simulink model "CPGPernaDireita"  (R2020a)
settings: Solver=VariableStepAuto  StartTime=0.0  StopTime=0.54  RelTol=1e-4
values from neighbouring files (symbols this model uses):
  b1 = 14.786    [CPG_PernaDireita_Parametros.m]
  b2 = b    (= 2.5)    [CPG_PernaDireita_Parametros.m]
  b3 = b    (= 2.5)    [CPG_PernaDireita_Parametros.m]
  b5 = b    (= 2.5)    [CPG_PernaDireita_Parametros.m]
  feed1 = 0    [CPG_PernaDireita_Parametros.m]
  feed10 = 0    [CPG_PernaDireita_Parametros.m]
  feed2 = 0    [CPG_PernaDireita_Parametros.m]
  feed3 = 0    [CPG_PernaDireita_Parametros.m]
  feed4 = 0    [CPG_PernaDireita_Parametros.m]
  feed5 = 0    [CPG_PernaDireita_Parametros.m]
  feed6 = 0    [CPG_PernaDireita_Parametros.m]
  feed9 = 0    [CPG_PernaDireita_Parametros.m]
  S1 = 50    [CPG_PernaDireita_Parametros.m]
  S2 = S0    (= 5)    [CPG_PernaDireita_Parametros.m]
  S3 = S0    (= 5)    [CPG_PernaDireita_Parametros.m]
  S5 = S0    (= 5)    [CPG_PernaDireita_Parametros.m]
  ta1 = 0.04    [CPG_PernaDireita_Parametros.m]
  ta10 = 0.3    [CPG_PernaDireita_Parametros.m]
  ta2 = 20    [CPG_PernaDireita_Parametros.m]
  ta3 = 0.6    [CPG_PernaDireita_Parametros.m]
  ta4 = 0.6    [CPG_PernaDireita_Parametros.m]
  ta5 = 0.3    [CPG_PernaDireita_Parametros.m]
  ta6 = 0.3    [CPG_PernaDireita_Parametros.m]
  ta9 = 0.3    [CPG_PernaDireita_Parametros.m]
  tr1 = 0.0004    [CPG_PernaDireita_Parametros.m]
  tr10 = 0.025    [CPG_PernaDireita_Parametros.m]
  tr2 = 0.1    [CPG_PernaDireita_Parametros.m]
  tr3 = 0.0005    [CPG_PernaDireita_Parametros.m]
  tr4 = 0.05    [CPG_PernaDireita_Parametros.m]
  tr5 = 0.025    [CPG_PernaDireita_Parametros.m]
  tr6 = 0.025    [CPG_PernaDireita_Parametros.m]
  tr9 = 0.025    [CPG_PernaDireita_Parametros.m]
  w10_1 = -1    [CPG_PernaDireita_Parametros.m]
  w10_2 = -1    [CPG_PernaDireita_Parametros.m]
  w10_5 = 0    [CPG_PernaDireita_Parametros.m]
  w10_6 = 0    [CPG_PernaDireita_Parametros.m]
  w10_9 = -2    [CPG_PernaDireita_Parametros.m]
  w12 = -2.64    [CPG_PernaDireita_Parametros.m]
  w13 = -1.7585    [CPG_PernaDireita_Parametros.m]
  w15 = 0    [CPG_PernaDireita_Parametros.m]
  w16 = 0    [CPG_PernaDireita_Parametros.m]
  w19 = 0    [CPG_PernaDireita_Parametros.m]
  w1_10 = 0    [CPG_PernaDireita_Parametros.m]
  w21 = -2    [CPG_PernaDireita_Parametros.m]
  w24 = -1    [CPG_PernaDireita_Parametros.m]
  w25 = 0    [CPG_PernaDireita_Parametros.m]
  w26 = 0    [CPG_PernaDireita_Parametros.m]
  w29 = 0    [CPG_PernaDireita_Parametros.m]
  w2_10 = 0    [CPG_PernaDireita_Parametros.m]
  w31 = -1    [CPG_PernaDireita_Parametros.m]
  w34 = -2    [CPG_PernaDireita_Parametros.m]
  w37 = 0    [CPG_PernaDireita_Parametros.m]
  w38 = 0    [CPG_PernaDireita_Parametros.m]
  w3_11 = 0    [CPG_PernaDireita_Parametros.m]
  w3_12 = 0    [CPG_PernaDireita_Parametros.m]
  w42 = -1    [CPG_PernaDireita_Parametros.m]
  w43 = -2    [CPG_PernaDireita_Parametros.m]
  w47 = 0    [CPG_PernaDireita_Parametros.m]
  w48 = 0    [CPG_PernaDireita_Parametros.m]
  w4_11 = 0    [CPG_PernaDireita_Parametros.m]
  w4_12 = 0    [CPG_PernaDireita_Parametros.m]
  w51 = 0    [CPG_PernaDireita_Parametros.m]
  w52 = 0    [CPG_PernaDireita_Parametros.m]
  w56 = -2    [CPG_PernaDireita_Parametros.m]
  w59 = 0    [CPG_PernaDireita_Parametros.m]
  w5_10 = 0    [CPG_PernaDireita_Parametros.m]
  w61 = -1    [CPG_PernaDireita_Parametros.m]
  w62 = -1    [CPG_PernaDireita_Parametros.m]
  w65 = -2    [CPG_PernaDireita_Parametros.m]
  w69 = 0    [CPG_PernaDireita_Parametros.m]
  w6_10 = 0    [CPG_PernaDireita_Parametros.m]
  w91 = 0    [CPG_PernaDireita_Parametros.m]
  w92 = 0    [CPG_PernaDireita_Parametros.m]
  w95 = -0.5    [CPG_PernaDireita_Parametros.m]
  w96 = -0.5    [CPG_PernaDireita_Parametros.m]
  w9_10 = -2    [CPG_PernaDireita_Parametros.m]
  ws1 = 1    [CPG_PernaDireita_Parametros.m]
  ws10 = 1    [CPG_PernaDireita_Parametros.m]
  ws2 = 1    [CPG_PernaDireita_Parametros.m]
  ws3 = 1    [CPG_PernaDireita_Parametros.m]
  ws4 = 1    [CPG_PernaDireita_Parametros.m]
  ws5 = 1    [CPG_PernaDireita_Parametros.m]
  ws6 = 1    [CPG_PernaDireita_Parametros.m]
  ws9 = 1    [CPG_PernaDireita_Parametros.m]
  y11 = 0    [CPG_PernaDireita_Parametros.m]
  y12 = 0    [CPG_PernaDireita_Parametros.m]
  y7 = 0    [CPG_PernaDireita_Parametros.m]
  y8 = 0    [CPG_PernaDireita_Parametros.m]
settings Model: Creator=LUIS IZQUIERDO C  LastModifiedBy=LUIS IZQUIERDO C
settings DataIOCC: DSMLogging=off  ReturnWorkspaceOutputsName=SDOSimTest_Log

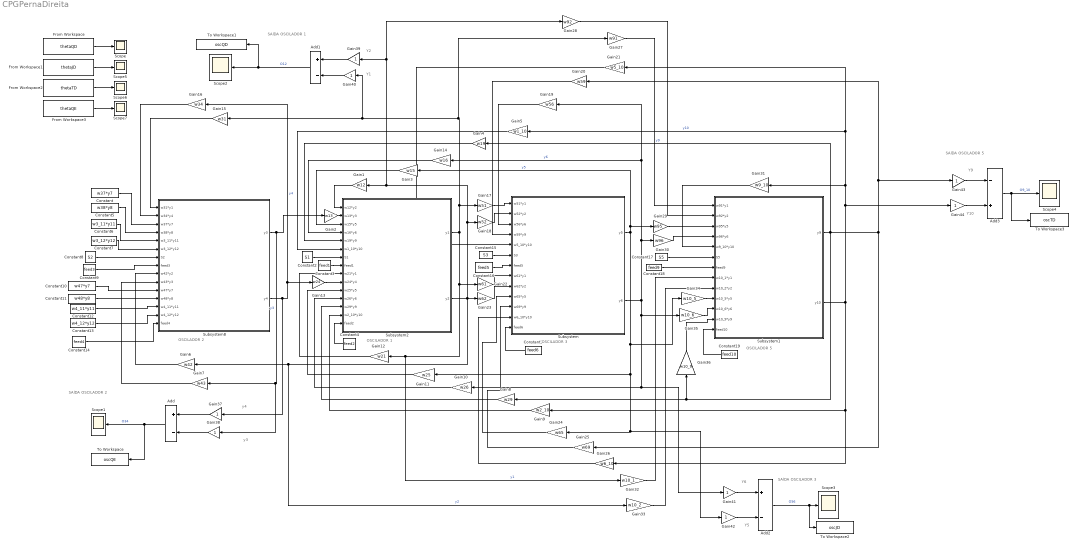
== system CPGPernaDireita ==
  note: OSCILADOR 1
  note: SAÍDA OSCILADOR 3
  note: y4
  note: SAÍDA OSCILADOR 2
  note: OSCILADOR 2
  note: OSCILADOR 5
  note: Y1
  note: Y6
  note: Y2
  note: SAÍDA OSCILADOR 1
  note: y3
  note: SAÍDA OSCILADOR 5
  note: Y5
  note: Y9
  note: OSCILADOR 3
  note: Y10
  Add : Sum  Inputs=+-
  Add1 : Sum  Inputs=+-
  Add2 : Sum  Inputs=+-
  Add3 : Sum  Inputs=-+
  Constant : Constant  Value=w37*y7
  Constant1 : Constant  Value=feed6
  Constant10 : Constant  Value=w47*y7
  Constant11 : Constant  Value=w48*y8
  Constant12 : Constant  Value=w4_11*y11
  Constant13 : Constant  Value=w4_12*y12
  Constant14 : Constant  Value=feed4
  Constant15 : Constant  Value=S3
  Constant16 : Constant  Value=feed5
  Constant17 : Constant  Value=S5
  Constant18 : Constant  Value=feed9
  Constant19 : Constant  Value=feed10
  Constant2 : Constant  Value=S1
  Constant3 : Constant  Value=feed1
  Constant4 : Constant  Value=feed2
  Constant5 : Constant  Value=w38*y8
  Constant6 : Constant  Value=w3_11*y11
  Constant7 : Constant  Value=w3_12*y12
  Constant8 : Constant  Value=S2
  Constant9 : Constant  Value=feed3
  From Workspace : FromWorkspace  VariableName=thetaQD  OutputAfterFinalValue=Holding final value
  From Workspace1 : FromWorkspace  VariableName=thetaJD  OutputAfterFinalValue=Holding final value
  From Workspace2 : FromWorkspace  VariableName=thetaTD  OutputAfterFinalValue=Holding final value
  From Workspace3 : FromWorkspace  VariableName=thetaQE  OutputAfterFinalValue=Holding final value
  Gain1 : Gain  Gain=w12
  Gain10 : Gain  Gain=w26
  Gain11 : Gain  Gain=w25
  Gain12 : Gain  Gain=w21
  Gain13 : Gain  Gain=w24
  Gain14 : Gain  Gain=w16
  Gain15 : Gain  Gain=w31
  Gain16 : Gain  Gain=w34
  Gain17 : Gain  Gain=w51
  Gain18 : Gain  Gain=w52
  Gain19 : Gain  Gain=w56
  Gain2 : Gain  Gain=w13
  Gain20 : Gain  Gain=w59
  Gain21 : Gain  Gain=w5_10
  Gain22 : Gain  Gain=w61
  Gain23 : Gain  Gain=w62
  Gain24 : Gain  Gain=w65
  Gain25 : Gain  Gain=w69
  Gain26 : Gain  Gain=w6_10
  Gain27 : Gain  Gain=w91
  Gain28 : Gain  Gain=w92
  Gain29 : Gain  Gain=w95
  Gain3 : Gain  Gain=w15
  Gain30 : Gain  Gain=w96
  Gain31 : Gain  Gain=w9_10
  Gain32 : Gain  Gain=w10_1
  Gain33 : Gain  Gain=w10_2
  Gain34 : Gain  Gain=w10_5
  Gain35 : Gain  Gain=w10_6
  Gain36 : Gain  Gain=w10_9
  Gain{37..44} (8 alike) : Gain
  Gain4 : Gain  Gain=w19
  Gain5 : Gain  Gain=w1_10
  Gain6 : Gain  Gain=w42
  Gain7 : Gain  Gain=w43
  Gain8 : Gain  Gain=w29
  Gain9 : Gain  Gain=w2_10
  Scope{,1..7} (8 alike) : Scope
  Subsystem : Subsystem
  Subsystem1 : Subsystem
  Subsystem2 : Subsystem
  Subsystem8 : Subsystem
  To Workspace : ToWorkspace  VariableName=oscQE  SaveFormat=Timeseries  SampleTime=-1
  To Workspace1 : ToWorkspace  VariableName=oscQD  SaveFormat=Timeseries  SampleTime=-1
  To Workspace2 : ToWorkspace  VariableName=oscJD  SaveFormat=Timeseries  SampleTime=-1
  To Workspace3 : ToWorkspace  VariableName=oscTD  SaveFormat=Timeseries  SampleTime=-1
  wires:
  Constant3/1 -> Subsystem2/8(feed1)
  Gain10/1 -> Subsystem2/12(w26*y6)
  Subsystem8/1(y3) -> Gain2/1, Gain38/1, Gain7/1  "y3"
  Gain38/1 -> Add/2
  Gain4/1 -> Subsystem2/5(w19*y9)
  Gain43/1 -> Add3/1
  Gain9/1 -> Subsystem2/14(w2_10*y10)
  Constant10/1 -> Subsystem8/11(w47*y7)
  Constant8/1 -> Subsystem8/7(S2)
  Constant16/1 -> Subsystem/7(feed5)
  Subsystem8/2(y4) -> Gain16/1, Gain13/1, Gain37/1  "y4"
  Constant12/1 -> Subsystem8/13(w4_11*y11)
  Constant9/1 -> Subsystem8/8(feed3)
  Constant15/1 -> Subsystem/6(S3)
  Constant5/1 -> Subsystem8/4(w38*y8)
  Gain13/1 -> Subsystem2/10(w24*y4)
  From Workspace3/1 -> Scope7/1
  Gain17/1 -> Subsystem/1(w51*y1)
  Constant11/1 -> Subsystem8/12(w48*y8)
  Constant2/1 -> Subsystem2/7(S1)
  Subsystem1/1(y9) -> Gain36/1, Gain8/1, Gain4/1, Gain20/1, Gain43/1, Gain25/1  "y9"
  Subsystem2/1(y1) -> Gain27/1, Gain40/1, Gain15/1, Gain17/1, Gain22/1, Gain32/1, Gain12/1  "y1"
  Gain23/1 -> Subsystem/9(w62*y2)
  Add3/1 -> To Workspace3/1, Scope4/1  "O9_10"
  Constant/1 -> Subsystem8/3(w37*y7)
  Gain1/1 -> Subsystem2/1(w12*y2)
  Gain14/1 -> Subsystem2/4(w16*y6)
  Gain34/1 -> Subsystem1/10(w10_5*y5)
  Add/1 -> To Workspace/1, Scope1/1  "O34"
  Constant19/1 -> Subsystem1/13(feed10)
  From Workspace/1 -> Scope/1
  From Workspace2/1 -> Scope6/1
  Gain2/1 -> Subsystem2/2(w13*y3)
  Gain6/1 -> Subsystem8/9(w42*y2)
  Constant4/1 -> Subsystem2/15(feed2)
  Gain24/1 -> Subsystem/10(w65*y5)
  Gain22/1 -> Subsystem/8(w61*y1)
  Gain36/1 -> Subsystem1/12(w10_9*y9)
  Gain15/1 -> Subsystem8/1(w31*y1)
  Constant7/1 -> Subsystem8/6(w3_12*y12)
  Gain26/1 -> Subsystem/12(w6_10*y10)
  Add2/1 -> To Workspace2/1, Scope3/1  "O56"
  Constant13/1 -> Subsystem8/14(w4_12*y12)
  Constant1/1 -> Subsystem/13(feed6)
  Gain40/1 -> Add1/2
  Gain25/1 -> Subsystem/11(w69*y9)
  Gain44/1 -> Add3/2
  Gain7/1 -> Subsystem8/10(w43*y3)
  Gain35/1 -> Subsystem1/11(w10_6*y6)
  Constant6/1 -> Subsystem8/5(w3_11*y11)
  Gain16/1 -> Subsystem8/2(w34*y4)
  Gain19/1 -> Subsystem/3(w56*y6)
  From Workspace1/1 -> Scope5/1
  Constant18/1 -> Subsystem1/7(feed9)
  Gain31/1 -> Subsystem1/5(w9_10*y10)
  Gain30/1 -> Subsystem1/4(w96*y6)
  Gain37/1 -> Add/1
  Constant17/1 -> Subsystem1/6(S5)
  Gain8/1 -> Subsystem2/13(w29*y9)
  Gain29/1 -> Subsystem1/3(w95*y5)
  Gain41/1 -> Add2/1
  Gain21/1 -> Subsystem/5(w5_10*y10)
  Subsystem/2(y6) -> Gain35/1, Gain10/1, Gain41/1, Gain30/1, Gain19/1, Gain14/1  "y6"
  Subsystem1/2(y10) -> Gain31/1, Gain5/1, Gain21/1, Gain44/1, Gain9/1, Gain26/1  "y10"
  Gain27/1 -> Subsystem1/1(w91*y1)
  Gain12/1 -> Subsystem2/9(w21*y1)
  Gain11/1 -> Subsystem2/11(w25*y5)
  Subsystem2/2(y2) -> Gain23/1, Gain33/1, Gain6/1, Gain18/1, Gain1/1, Gain39/1, Gain28/1  "y2"
  Gain28/1 -> Subsystem1/2(w92*y2)
  Gain42/1 -> Add2/2
  Gain18/1 -> Subsystem/2(w52*y2)
  Subsystem/1(y5) -> Gain34/1, Gain42/1, Gain24/1, Gain11/1, Gain29/1, Gain3/1  "y5"
  Gain33/1 -> Subsystem1/9(w10_2*y2)
  Gain32/1 -> Subsystem1/8(w10_1*y1)
  Gain5/1 -> Subsystem2/6(w1_10*y10)
  Gain20/1 -> Subsystem/4(w59*y9)
  Constant14/1 -> Subsystem8/15(feed4)
  Gain39/1 -> Add1/1
  Gain3/1 -> Subsystem2/3(w15*y5)
  Add1/1 -> To Workspace1/1, Scope2/1  "O12"

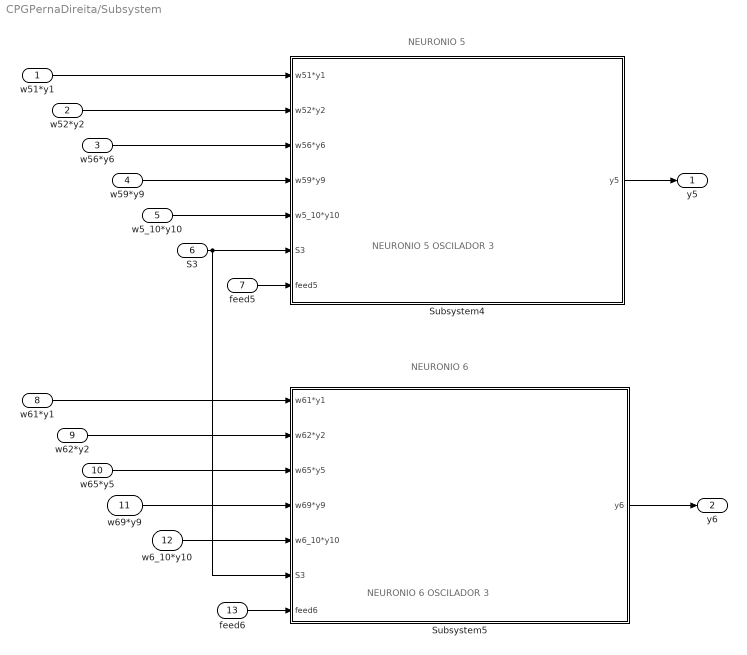
== system CPGPernaDireita/Subsystem ==
  note: NEURONIO 6
  note: NEURONIO 5
  note: NEURONIO 6 OSCILADOR 3
  note: NEURONIO 5 OSCILADOR 3
  w51*y1 : Inport
  w52*y2 : Inport  Port=2
  w56*y6 : Inport  Port=3
  w59*y9 : Inport  Port=4
  w5_10*y10 : Inport  Port=5
  S3 : Inport  Port=6
  feed5 : Inport  Port=7
  w61*y1 : Inport  Port=8
  w62*y2 : Inport  Port=9
  w65*y5 : Inport  Port=10
  w69*y9 : Inport  Port=11
  w6_10*y10 : Inport  Port=12
  feed6 : Inport  Port=13
  Subsystem4 : Subsystem
  Subsystem5 : Subsystem
  y5 : Outport  VectorParamsAs1DForOutWhenUnconnected=off
  y6 : Outport  Port=2  VectorParamsAs1DForOutWhenUnconnected=off
  wires:
  w56*y6/1 -> Subsystem4/3(w56*y6)
  feed5/1 -> Subsystem4/7(feed5)
  w59*y9/1 -> Subsystem4/4(w59*y9)
  w62*y2/1 -> Subsystem5/2(w62*y2)
  w6_10*y10/1 -> Subsystem5/5(w6_10*y10)
  w69*y9/1 -> Subsystem5/4(w69*y9)
  w5_10*y10/1 -> Subsystem4/5(w5_10*y10)
  w61*y1/1 -> Subsystem5/1(w61*y1)
  w65*y5/1 -> Subsystem5/3(w65*y5)
  Subsystem5/1(y6) -> y6/1
  w51*y1/1 -> Subsystem4/1(w51*y1)
  w52*y2/1 -> Subsystem4/2(w52*y2)
  S3/1 -> Subsystem5/6(S3), Subsystem4/6(S3)
  Subsystem4/1(y5) -> y5/1
  feed6/1 -> Subsystem5/7(feed6)

== system CPGPernaDireita/Subsystem1 ==
  note: NEURONIO 10
  note: NEURONIO 9
  note: NEURONIO 10 OSCILADOR 5
  note: NEURONIO 9 OSCILADOR 5
  w91*y1 : Inport
  w92*y2 : Inport  Port=2
  w95*y5 : Inport  Port=3
  w96*y6 : Inport  Port=4
  w9_10*y10 : Inport  Port=5
  S5 : Inport  Port=6
  feed9 : Inport  Port=7
  w10_1*y1 : Inport  Port=8
  w10_2*y2 : Inport  Port=9
  w10_5*y5 : Inport  Port=10
  w10_6*y6 : Inport  Port=11
  w10_9*y9 : Inport  Port=12
  feed10 : Inport  Port=13
  Subsystem6 : Subsystem
  Subsystem7 : Subsystem
  y9 : Outport  VectorParamsAs1DForOutWhenUnconnected=off
  y10 : Outport  Port=2  VectorParamsAs1DForOutWhenUnconnected=off
  wires:
  Subsystem7/1(y10) -> y10/1
  w10_1*y1/1 -> Subsystem7/1(w10_1*y1)
  w10_2*y2/1 -> Subsystem7/2(w10_2*y2)
  Subsystem6/1(y9) -> y9/1
  feed10/1 -> Subsystem7/7(feed10)
  w10_5*y5/1 -> Subsystem7/3(w10_5*y5)
  feed9/1 -> Subsystem6/7(feed9)
  S5/1 -> Subsystem7/6(S5), Subsystem6/6(S5)
  w92*y2/1 -> Subsystem6/2(w92*y2)
  w10_9*y9/1 -> Subsystem7/5(w10_9*y9)
  w10_6*y6/1 -> Subsystem7/4(w10_6*y6)
  w91*y1/1 -> Subsystem6/1(w91*y1)
  w95*y5/1 -> Subsystem6/3(w95*y5)
  w96*y6/1 -> Subsystem6/4(w96*y6)
  w9_10*y10/1 -> Subsystem6/5(w9_10*y10)

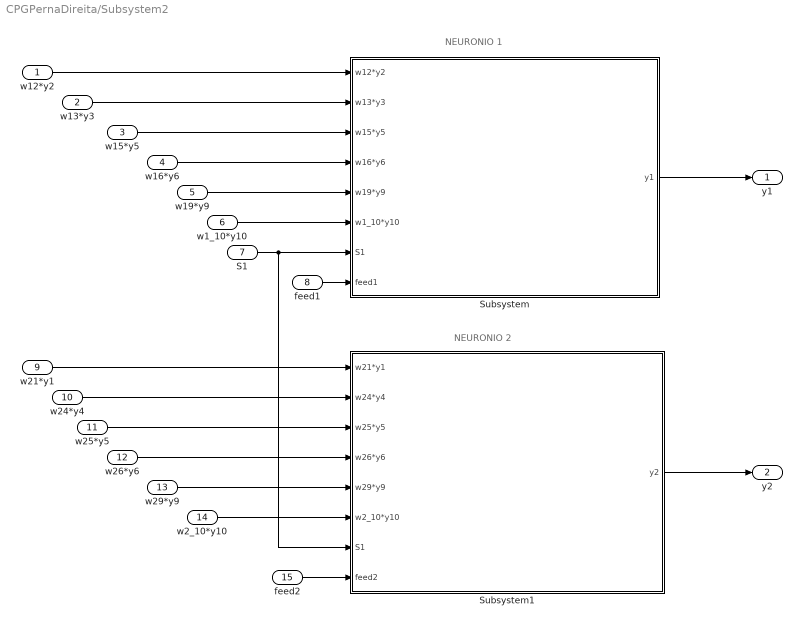
== system CPGPernaDireita/Subsystem2 ==
  note: NEURONIO 1
  note: NEURONIO 2
  w12*y2 : Inport
  w13*y3 : Inport  Port=2
  w15*y5 : Inport  Port=3
  w16*y6 : Inport  Port=4
  w19*y9 : Inport  Port=5
  w1_10*y10 : Inport  Port=6
  S1 : Inport  Port=7
  feed1 : Inport  Port=8
  w21*y1 : Inport  Port=9
  w24*y4 : Inport  Port=10
  w25*y5 : Inport  Port=11
  w26*y6 : Inport  Port=12
  w29*y9 : Inport  Port=13
  w2_10*y10 : Inport  Port=14
  feed2 : Inport  Port=15
  Subsystem : Subsystem
  Subsystem1 : Subsystem
  y1 : Outport  VectorParamsAs1DForOutWhenUnconnected=off
  y2 : Outport  Port=2  VectorParamsAs1DForOutWhenUnconnected=off
  wires:
  w16*y6/1 -> Subsystem/4(w16*y6)
  w21*y1/1 -> Subsystem1/1(w21*y1)
  w15*y5/1 -> Subsystem/3(w15*y5)
  w12*y2/1 -> Subsystem/1(w12*y2)
  w19*y9/1 -> Subsystem/5(w19*y9)
  w13*y3/1 -> Subsystem/2(w13*y3)
  w1_10*y10/1 -> Subsystem/6("w1_10*y10 ")
  feed1/1 -> Subsystem/8(feed1)
  w26*y6/1 -> Subsystem1/4(w26*y6)
  w24*y4/1 -> Subsystem1/2(w24*y4)
  w25*y5/1 -> Subsystem1/3(w25*y5)
  S1/1 -> Subsystem1/7(S1), Subsystem/7(S1)
  w29*y9/1 -> Subsystem1/5(w29*y9)
  w2_10*y10/1 -> Subsystem1/6("w2_10*y10 ")
  feed2/1 -> Subsystem1/8(feed2)
  Subsystem/1(y1) -> y1/1
  Subsystem1/1(y2) -> y2/1

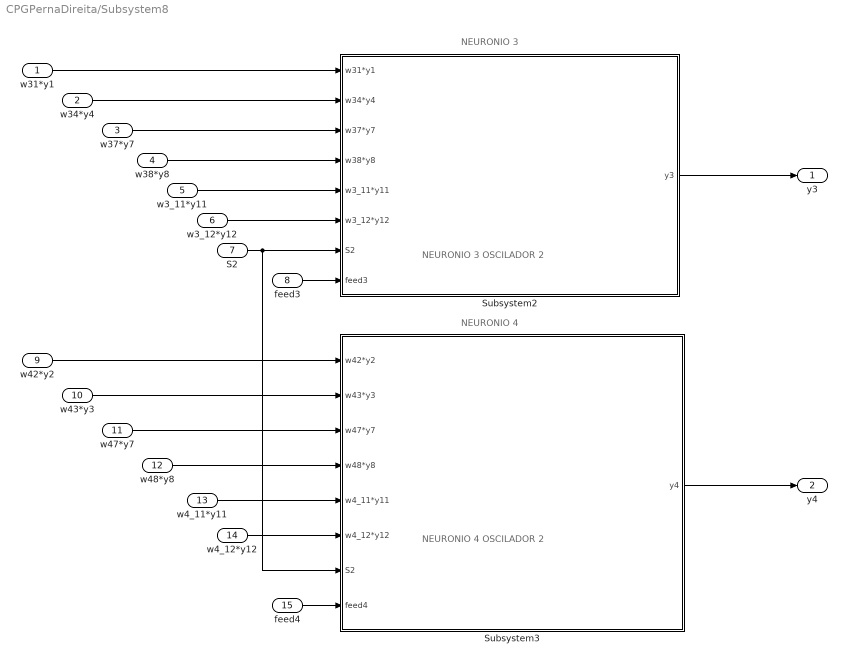
== system CPGPernaDireita/Subsystem8 ==
  note: NEURONIO 4
  note: NEURONIO 3
  note: NEURONIO 3 OSCILADOR 2
  note: NEURONIO 4 OSCILADOR 2
  w31*y1 : Inport
  w34*y4 : Inport  Port=2
  w37*y7 : Inport  Port=3
  w38*y8 : Inport  Port=4
  w3_11*y11 : Inport  Port=5
  w3_12*y12 : Inport  Port=6
  S2 : Inport  Port=7
  feed3 : Inport  Port=8
  w42*y2 : Inport  Port=9
  w43*y3 : Inport  Port=10
  w47*y7 : Inport  Port=11
  w48*y8 : Inport  Port=12
  w4_11*y11 : Inport  Port=13
  w4_12*y12 : Inport  Port=14
  feed4 : Inport  Port=15
  Subsystem2 : Subsystem
  Subsystem3 : Subsystem
  y3 : Outport  VectorParamsAs1DForOutWhenUnconnected=off
  y4 : Outport  Port=2  VectorParamsAs1DForOutWhenUnconnected=off
  wires:
  feed4/1 -> Subsystem3/8(feed4)
  feed3/1 -> Subsystem2/8(feed3)
  w4_12*y12/1 -> Subsystem3/6("w4_12*y12 ")
  w4_11*y11/1 -> Subsystem3/5(w4_11*y11)
  w42*y2/1 -> Subsystem3/1(w42*y2)
  w34*y4/1 -> Subsystem2/2(w34*y4)
  w43*y3/1 -> Subsystem3/2(w43*y3)
  w37*y7/1 -> Subsystem2/3(w37*y7)
  w31*y1/1 -> Subsystem2/1(w31*y1)
  w38*y8/1 -> Subsystem2/4(w38*y8)
  w3_12*y12/1 -> Subsystem2/6("w3_12*y12 ")
  Subsystem2/1(y3) -> y3/1
  w3_11*y11/1 -> Subsystem2/5(w3_11*y11)
  S2/1 -> Subsystem3/7(S2), Subsystem2/7(S2)
  w47*y7/1 -> Subsystem3/3(w47*y7)
  w48*y8/1 -> Subsystem3/4(w48*y8)
  Subsystem3/1(y4) -> y4/1

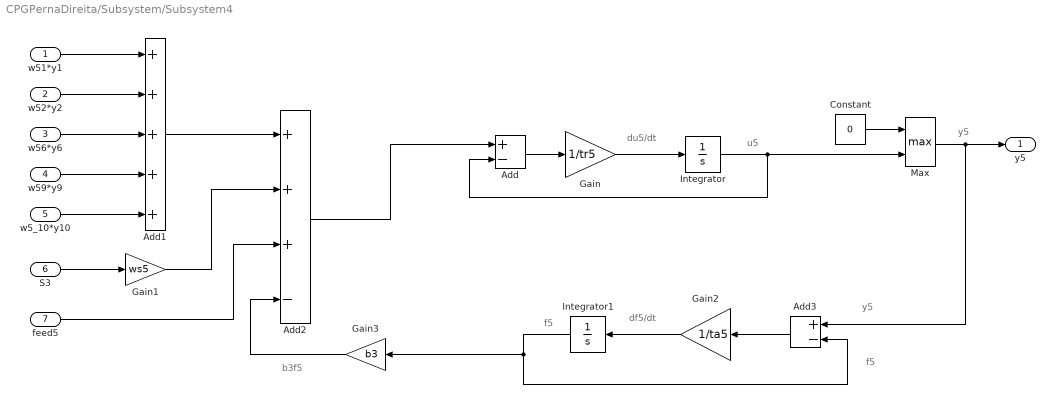
== system CPGPernaDireita/Subsystem/Subsystem4 ==
  note: b3f5
  note: y5
  note: y5
  note: f5
  note: u5
  note: du5/dt
  note: df5/dt
  note: f5
  w51*y1 : Inport
  w52*y2 : Inport  Port=2
  w56*y6 : Inport  Port=3
  w59*y9 : Inport  Port=4
  w5_10*y10 : Inport  Port=5
  S3 : Inport  Port=6
  feed5 : Inport  Port=7
  Add : Sum  Inputs=+-
  Add1 : Sum  Inputs=+++++
  Add2 : Sum  Inputs=+++-
  Add3 : Sum  Inputs=+-
  Constant : Constant  Value=0
  Gain : Gain  Gain=1/tr5
  Gain1 : Gain  Gain=ws5
  Gain2 : Gain  Gain=1/ta5
  Gain3 : Gain  Gain=b3
  Integrator : Integrator
  Integrator1 : Integrator
  Max : MinMax  Function=max  Inputs=2
  y5 : Outport  VectorParamsAs1DForOutWhenUnconnected=off
  wires:
  w52*y2/1 -> Add1/2
  Add2/1 -> Add/1
  Add3/1 -> Gain2/1
  w56*y6/1 -> Add1/3
  Add/1 -> Gain/1
  Integrator1/1 -> Gain3/1, Add3/2
  Max/1 -> y5/1, Add3/1
  Constant/1 -> Max/1
  feed5/1 -> Add2/3
  Gain1/1 -> Add2/2
  w51*y1/1 -> Add1/1
  Gain2/1 -> Integrator1/1
  Add1/1 -> Add2/1
  Integrator/1 -> Add/2, Max/2
  Gain/1 -> Integrator/1
  S3/1 -> Gain1/1
  Gain3/1 -> Add2/4
  w59*y9/1 -> Add1/4
  w5_10*y10/1 -> Add1/5

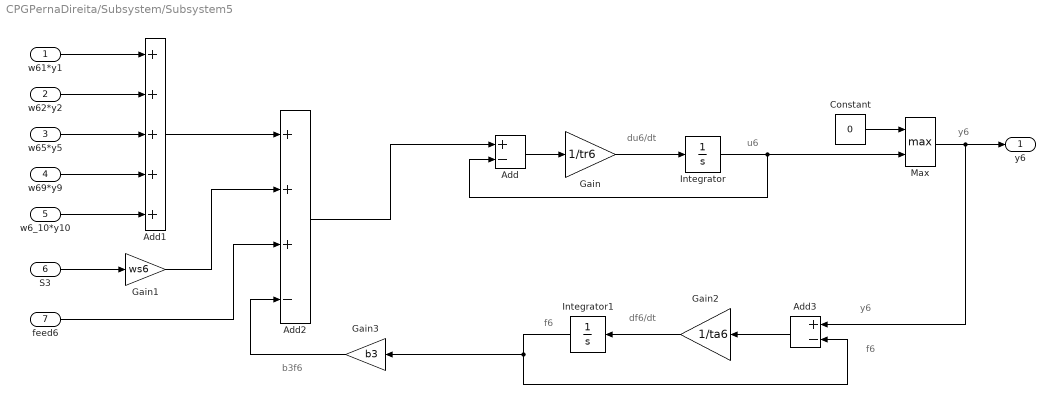
== system CPGPernaDireita/Subsystem/Subsystem5 ==
  note: b3f6
  note: y6
  note: y6
  note: f6
  note: u6
  note: du6/dt
  note: df6/dt
  note: f6
  w61*y1 : Inport
  w62*y2 : Inport  Port=2
  w65*y5 : Inport  Port=3
  w69*y9 : Inport  Port=4
  w6_10*y10 : Inport  Port=5
  S3 : Inport  Port=6
  feed6 : Inport  Port=7
  Add : Sum  Inputs=+-
  Add1 : Sum  Inputs=+++++
  Add2 : Sum  Inputs=+++-
  Add3 : Sum  Inputs=+-
  Constant : Constant  Value=0
  Gain : Gain  Gain=1/tr6
  Gain1 : Gain  Gain=ws6
  Gain2 : Gain  Gain=1/ta6
  Gain3 : Gain  Gain=b3
  Integrator : Integrator
  Integrator1 : Integrator
  Max : MinMax  Function=max  Inputs=2
  y6 : Outport  VectorParamsAs1DForOutWhenUnconnected=off
  wires:
  w62*y2/1 -> Add1/2
  Add2/1 -> Add/1
  Add3/1 -> Gain2/1
  w65*y5/1 -> Add1/3
  Add/1 -> Gain/1
  Integrator1/1 -> Gain3/1, Add3/2
  Max/1 -> y6/1, Add3/1
  Constant/1 -> Max/1
  feed6/1 -> Add2/3
  Gain1/1 -> Add2/2
  w61*y1/1 -> Add1/1
  Gain2/1 -> Integrator1/1
  Add1/1 -> Add2/1
  Integrator/1 -> Add/2, Max/2
  Gain/1 -> Integrator/1
  S3/1 -> Gain1/1
  Gain3/1 -> Add2/4
  w69*y9/1 -> Add1/4
  w6_10*y10/1 -> Add1/5

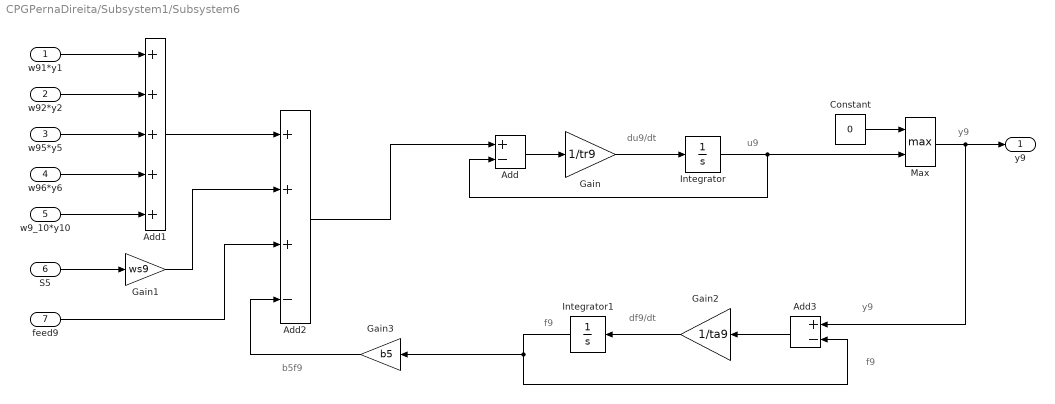
== system CPGPernaDireita/Subsystem1/Subsystem6 ==
  note: b5f9
  note: y9
  note: y9
  note: f9
  note: u9
  note: du9/dt
  note: df9/dt
  note: f9
  w91*y1 : Inport
  w92*y2 : Inport  Port=2
  w95*y5 : Inport  Port=3
  w96*y6 : Inport  Port=4
  w9_10*y10 : Inport  Port=5
  S5 : Inport  Port=6
  feed9 : Inport  Port=7
  Add : Sum  Inputs=+-
  Add1 : Sum  Inputs=+++++
  Add2 : Sum  Inputs=+++-
  Add3 : Sum  Inputs=+-
  Constant : Constant  Value=0
  Gain : Gain  Gain=1/tr9
  Gain1 : Gain  Gain=ws9
  Gain2 : Gain  Gain=1/ta9
  Gain3 : Gain  Gain=b5
  Integrator : Integrator
  Integrator1 : Integrator
  Max : MinMax  Function=max  Inputs=2
  y9 : Outport  VectorParamsAs1DForOutWhenUnconnected=off
  wires:
  w92*y2/1 -> Add1/2
  Add2/1 -> Add/1
  Add3/1 -> Gain2/1
  w95*y5/1 -> Add1/3
  Add/1 -> Gain/1
  Integrator1/1 -> Gain3/1, Add3/2
  Max/1 -> y9/1, Add3/1
  Constant/1 -> Max/1
  feed9/1 -> Add2/3
  Gain1/1 -> Add2/2
  w91*y1/1 -> Add1/1
  Gain2/1 -> Integrator1/1
  Add1/1 -> Add2/1
  Integrator/1 -> Add/2, Max/2
  Gain/1 -> Integrator/1
  S5/1 -> Gain1/1
  Gain3/1 -> Add2/4
  w96*y6/1 -> Add1/4
  w9_10*y10/1 -> Add1/5

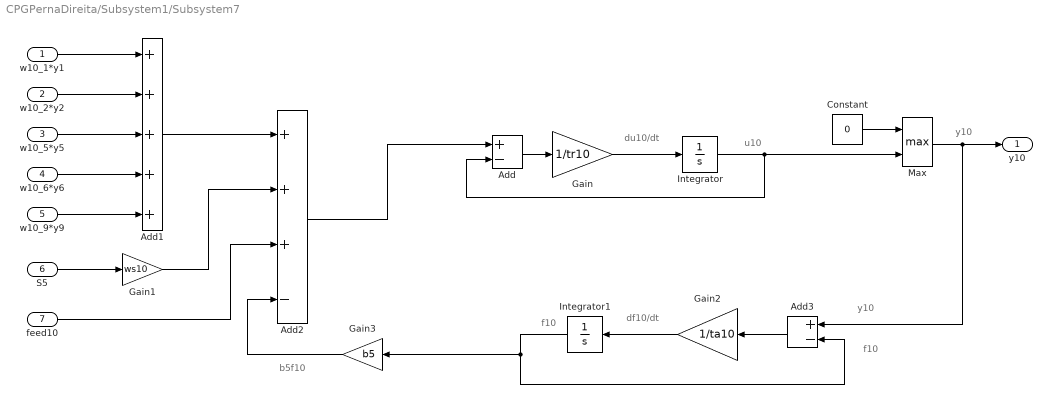
== system CPGPernaDireita/Subsystem1/Subsystem7 ==
  note: b5f10
  note: y10
  note: y10
  note: f10
  note: u10
  note: du10/dt
  note: df10/dt
  note: f10
  w10_1*y1 : Inport
  w10_2*y2 : Inport  Port=2
  w10_5*y5 : Inport  Port=3
  w10_6*y6 : Inport  Port=4
  w10_9*y9 : Inport  Port=5
  S5 : Inport  Port=6
  feed10 : Inport  Port=7
  Add : Sum  Inputs=+-
  Add1 : Sum  Inputs=+++++
  Add2 : Sum  Inputs=+++-
  Add3 : Sum  Inputs=+-
  Constant : Constant  Value=0
  Gain : Gain  Gain=1/tr10
  Gain1 : Gain  Gain=ws10
  Gain2 : Gain  Gain=1/ta10
  Gain3 : Gain  Gain=b5
  Integrator : Integrator
  Integrator1 : Integrator
  Max : MinMax  Function=max  Inputs=2
  y10 : Outport  VectorParamsAs1DForOutWhenUnconnected=off
  wires:
  w10_2*y2/1 -> Add1/2
  Add2/1 -> Add/1
  Add3/1 -> Gain2/1
  w10_5*y5/1 -> Add1/3
  Add/1 -> Gain/1
  Integrator1/1 -> Gain3/1, Add3/2
  Max/1 -> y10/1, Add3/1
  Constant/1 -> Max/1
  feed10/1 -> Add2/3
  Gain1/1 -> Add2/2
  w10_1*y1/1 -> Add1/1
  Gain2/1 -> Integrator1/1
  Add1/1 -> Add2/1
  Integrator/1 -> Add/2, Max/2
  Gain/1 -> Integrator/1
  S5/1 -> Gain1/1
  Gain3/1 -> Add2/4
  w10_6*y6/1 -> Add1/4
  w10_9*y9/1 -> Add1/5

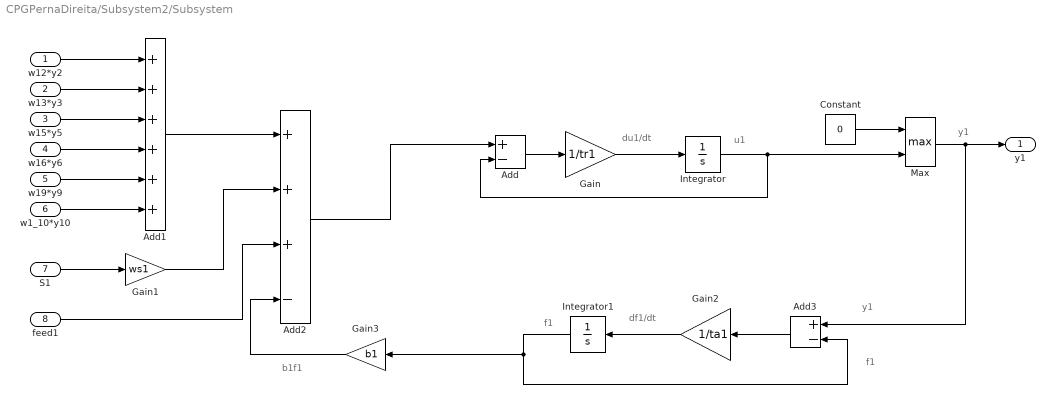
== system CPGPernaDireita/Subsystem2/Subsystem ==
  note: b1f1
  note: y1
  note: y1
  note: f1
  note: u1
  note: du1/dt
  note: df1/dt
  note: f1
  w12*y2 : Inport
  w13*y3 : Inport  Port=2
  w15*y5 : Inport  Port=3
  w16*y6 : Inport  Port=4
  w19*y9 : Inport  Port=5
  "w1_10*y10 " : Inport  Port=6
  S1 : Inport  Port=7
  feed1 : Inport  Port=8
  Add : Sum  Inputs=+-
  Add1 : Sum  Inputs=++++++
  Add2 : Sum  Inputs=+++-
  Add3 : Sum  Inputs=+-
  Constant : Constant  Value=0
  Gain : Gain  Gain=1/tr1
  Gain1 : Gain  Gain=ws1
  Gain2 : Gain  Gain=1/ta1
  Gain3 : Gain  Gain=b1
  Integrator : Integrator
  Integrator1 : Integrator
  Max : MinMax  Function=max  Inputs=2
  y1 : Outport  VectorParamsAs1DForOutWhenUnconnected=off
  wires:
  w13*y3/1 -> Add1/2
  Add2/1 -> Add/1
  Add3/1 -> Gain2/1
  w15*y5/1 -> Add1/3
  Add/1 -> Gain/1
  Integrator1/1 -> Gain3/1, Add3/2
  Max/1 -> y1/1, Add3/1
  Constant/1 -> Max/1
  feed1/1 -> Add2/3
  Gain1/1 -> Add2/2
  w12*y2/1 -> Add1/1
  Gain2/1 -> Integrator1/1
  Add1/1 -> Add2/1
  Integrator/1 -> Add/2, Max/2
  Gain/1 -> Integrator/1
  S1/1 -> Gain1/1
  Gain3/1 -> Add2/4
  w16*y6/1 -> Add1/4
  w19*y9/1 -> Add1/5
  "w1_10*y10 "/1 -> Add1/6

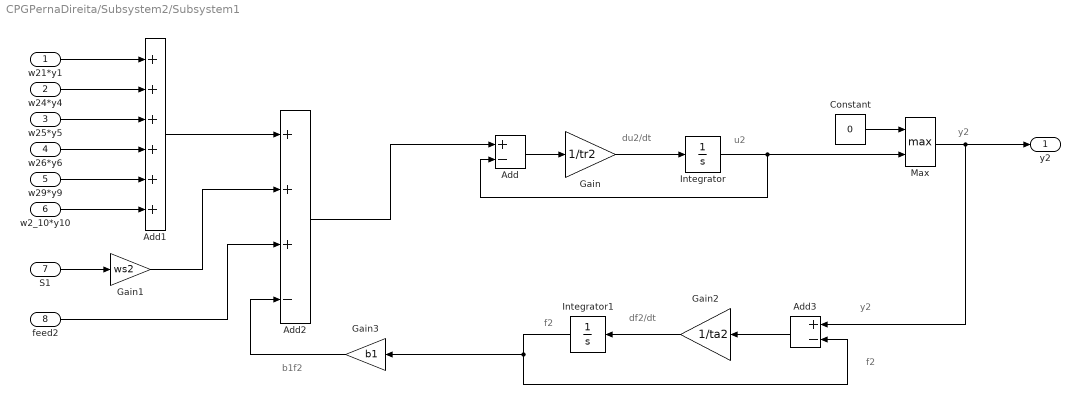
== system CPGPernaDireita/Subsystem2/Subsystem1 ==
  note: b1f2
  note: y2
  note: y2
  note: f2
  note: u2
  note: du2/dt
  note: df2/dt
  note: f2
  w21*y1 : Inport
  w24*y4 : Inport  Port=2
  w25*y5 : Inport  Port=3
  w26*y6 : Inport  Port=4
  w29*y9 : Inport  Port=5
  "w2_10*y10 " : Inport  Port=6
  S1 : Inport  Port=7
  feed2 : Inport  Port=8
  Add : Sum  Inputs=+-
  Add1 : Sum  Inputs=++++++
  Add2 : Sum  Inputs=+++-
  Add3 : Sum  Inputs=+-
  Constant : Constant  Value=0
  Gain : Gain  Gain=1/tr2
  Gain1 : Gain  Gain=ws2
  Gain2 : Gain  Gain=1/ta2
  Gain3 : Gain  Gain=b1
  Integrator : Integrator
  Integrator1 : Integrator
  Max : MinMax  Function=max  Inputs=2
  y2 : Outport  VectorParamsAs1DForOutWhenUnconnected=off
  wires:
  w24*y4/1 -> Add1/2
  Add2/1 -> Add/1
  Add3/1 -> Gain2/1
  w25*y5/1 -> Add1/3
  Add/1 -> Gain/1
  Integrator1/1 -> Gain3/1, Add3/2
  Max/1 -> y2/1, Add3/1
  Constant/1 -> Max/1
  feed2/1 -> Add2/3
  Gain1/1 -> Add2/2
  w21*y1/1 -> Add1/1
  Gain2/1 -> Integrator1/1
  Add1/1 -> Add2/1
  Integrator/1 -> Add/2, Max/2
  Gain/1 -> Integrator/1
  S1/1 -> Gain1/1
  Gain3/1 -> Add2/4
  w26*y6/1 -> Add1/4
  w29*y9/1 -> Add1/5
  "w2_10*y10 "/1 -> Add1/6

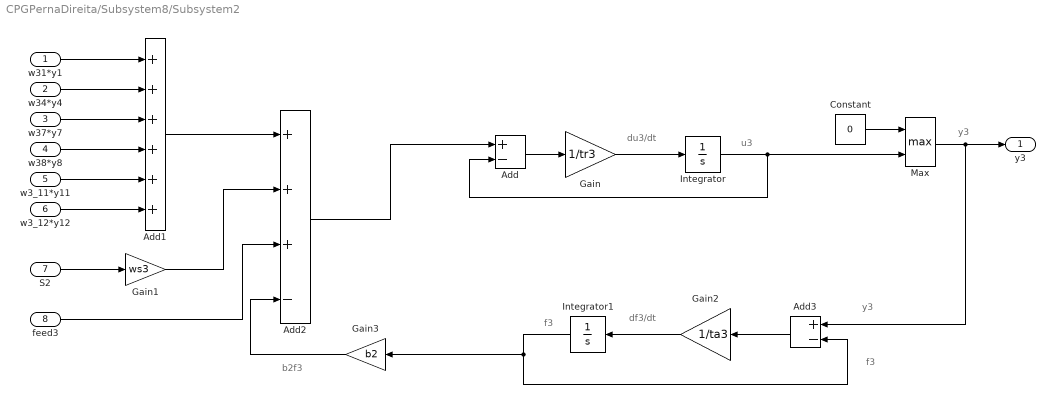
== system CPGPernaDireita/Subsystem8/Subsystem2 ==
  note: b2f3
  note: y3
  note: y3
  note: f3
  note: u3
  note: du3/dt
  note: df3/dt
  note: f3
  w31*y1 : Inport
  w34*y4 : Inport  Port=2
  w37*y7 : Inport  Port=3
  w38*y8 : Inport  Port=4
  w3_11*y11 : Inport  Port=5
  "w3_12*y12 " : Inport  Port=6
  S2 : Inport  Port=7
  feed3 : Inport  Port=8
  Add : Sum  Inputs=+-
  Add1 : Sum  Inputs=++++++
  Add2 : Sum  Inputs=+++-
  Add3 : Sum  Inputs=+-
  Constant : Constant  Value=0
  Gain : Gain  Gain=1/tr3
  Gain1 : Gain  Gain=ws3
  Gain2 : Gain  Gain=1/ta3
  Gain3 : Gain  Gain=b2
  Integrator : Integrator
  Integrator1 : Integrator
  Max : MinMax  Function=max  Inputs=2
  y3 : Outport  VectorParamsAs1DForOutWhenUnconnected=off
  wires:
  w34*y4/1 -> Add1/2
  Add2/1 -> Add/1
  Add3/1 -> Gain2/1
  w37*y7/1 -> Add1/3
  Add/1 -> Gain/1
  Integrator1/1 -> Gain3/1, Add3/2
  Max/1 -> y3/1, Add3/1
  Constant/1 -> Max/1
  feed3/1 -> Add2/3
  Gain1/1 -> Add2/2
  w31*y1/1 -> Add1/1
  Gain2/1 -> Integrator1/1
  Add1/1 -> Add2/1
  Integrator/1 -> Add/2, Max/2
  Gain/1 -> Integrator/1
  S2/1 -> Gain1/1
  Gain3/1 -> Add2/4
  w38*y8/1 -> Add1/4
  w3_11*y11/1 -> Add1/5
  "w3_12*y12 "/1 -> Add1/6

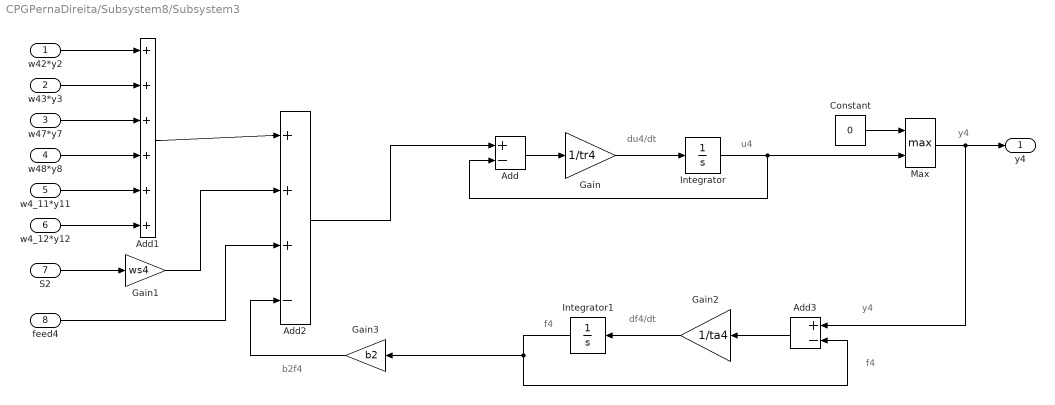
== system CPGPernaDireita/Subsystem8/Subsystem3 ==
  note: b2f4
  note: y4
  note: y4
  note: f4
  note: u4
  note: du4/dt
  note: df4/dt
  note: f4
  w42*y2 : Inport
  w43*y3 : Inport  Port=2
  w47*y7 : Inport  Port=3
  w48*y8 : Inport  Port=4
  w4_11*y11 : Inport  Port=5
  "w4_12*y12 " : Inport  Port=6
  S2 : Inport  Port=7
  feed4 : Inport  Port=8
  Add : Sum  Inputs=+-
  Add1 : Sum  Inputs=++++++
  Add2 : Sum  Inputs=+++-
  Add3 : Sum  Inputs=+-
  Constant : Constant  Value=0
  Gain : Gain  Gain=1/tr4
  Gain1 : Gain  Gain=ws4
  Gain2 : Gain  Gain=1/ta4
  Gain3 : Gain  Gain=b2
  Integrator : Integrator
  Integrator1 : Integrator
  Max : MinMax  Function=max  Inputs=2
  y4 : Outport  VectorParamsAs1DForOutWhenUnconnected=off
  wires:
  w43*y3/1 -> Add1/2
  Add2/1 -> Add/1
  Add3/1 -> Gain2/1
  w47*y7/1 -> Add1/3
  Add/1 -> Gain/1
  Integrator1/1 -> Gain3/1, Add3/2
  Max/1 -> y4/1, Add3/1
  Constant/1 -> Max/1
  feed4/1 -> Add2/3
  Gain1/1 -> Add2/2
  w42*y2/1 -> Add1/1
  Gain2/1 -> Integrator1/1
  Add1/1 -> Add2/1
  Integrator/1 -> Add/2, Max/2
  Gain/1 -> Integrator/1
  S2/1 -> Gain1/1
  Gain3/1 -> Add2/4
  w48*y8/1 -> Add1/4
  w4_11*y11/1 -> Add1/5
  "w4_12*y12 "/1 -> Add1/6
